simulink model "Aufgabe_13_simulink"  (Simulink 9.2)
settings: Solver=ode45  StartTime=0.0  StopTime=30  RelTol=1e-3  EnableMultiTasking=on
InitFcn:
  | Aufgabe_5_initFunction_Vorlage
StopFcn:
  | if Testen == 1
  | 
  | addpath('Check');
  | Aufgabe_5_Kontrolle;
  | 
  | end
undefined symbols (not defined in the file or in its folder): t_save
libraries: dspnetwork x4
settings Model: Creator=St  LastModifiedBy=danial
settings SolverCC: ZeroCrossAlgorithm=Adaptive
settings DataIOCC: SignalLoggingSaveFormat=Dataset
settings DebuggingCC: SolverPrmCheckMsg=warning  FcnCallInpInsideContextMsg=error
settings GRTTargetCC: CombineOutputUpdateFcns=on  GRTInterface=off
settings ConfigComp: CovSFcnEnable=off
settings CustomProperty: DataType=string  Value=0

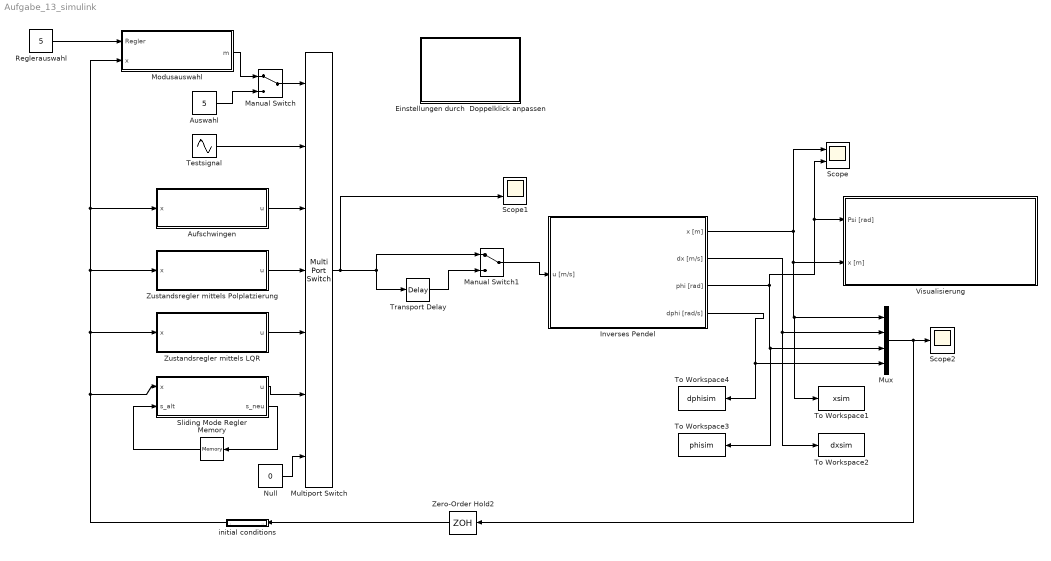
== system Aufgabe_13_simulink ==
  Aufschwingen : MATLAB Function  TreatAsAtomicUnit=on
  Auswahl : Constant  Value=5  SampleTime=-1
  Einstellungen durch  Doppelklick anpassen : MATLAB Function  InitFcn=tic  TreatAsAtomicUnit=on  mask{Auswahl=Bearbeiten}
      mask init:
      | maskStr = get_param(gcb,'Auswahl');
      | 
      | if strcmp(maskStr(1),'I')
      |      assignin('base','Testen',0)
      | else if strcmp(maskStr(1),'M')
      |         assignin('base','Testen',1)
      |     else
      |         assignin('base','Testen',2)
      |     end
      | end
  Inverses Pendel : Subsystem  TreatAsAtomicUnit=on  mask{x0=0, dx0=0.5, phi0=0, dphi0=0}
      mask prompts: x0 "Startposition Wagen [m]"; dx0 "Startgeschwindigkeit Wagen [m/s]"; phi0 "Startwinkel Pendel [rad]"; dphi0 "Startwinkelgeschwindigkeit Pendel [rad/s]"
  Manual Switch : ManualSwitch
  Manual Switch1 : ManualSwitch
  Memory : Memory  InitialCondition=-2
  Modusauswahl : MATLAB Function  TreatAsAtomicUnit=on
  Multiport Switch : MultiPortSwitch  Inputs=5  DataPortForDefault=Additional data port  DiagnosticForDefault=Warning
  Mux : Mux
  Null : Constant  Value=0  SampleTime=-1
  Reglerauswahl : Constant  Value=5  SampleTime=-1
  Scope : Scope  NumInputPorts=2
  Scope1 : Scope  NumInputPorts=2
  Scope2 : Scope
  Sliding Mode Regler : MATLAB Function  TreatAsAtomicUnit=on
  Testsignal : Sin  Amplitude=0.5  Frequency=6  SampleTime=0
  To Workspace1 : ToWorkspace  VariableName=xsim  SampleTime=t_save
  To Workspace2 : ToWorkspace  VariableName=dxsim  SampleTime=t_save
  To Workspace3 : ToWorkspace  VariableName=phisim  SampleTime=t_save
  To Workspace4 : ToWorkspace  VariableName=dphisim  SampleTime=t_save
  Transport Delay : TransportDelay  DelayTime=0.03
  Visualisierung : Subsystem
      mask init:
      | l_s = 0.5;              % Schienenlänge [m]
      settings: OpenFcn=|
      | !Pendel_Visualisierung_64bit\Pendel.blend.exe
      | !Pendel_Visualisierung_32bit\Pendel.blend.exe
  Zero-Order Hold2 : ZeroOrderHold  SampleTime=0.005
  Zustandsregler mittels LQR : MATLAB Function  TreatAsAtomicUnit=on
  Zustandsregler mittels Polplatzierung : MATLAB Function  TreatAsAtomicUnit=on
  initial conditions : Subsystem  mask{x0=0, dx0=0, phi0=pi, dphi0=0}
      mask prompts: x0 "Startposition Wagen [m]"; dx0 "Startgeschwindigkeit Wagen [m/s]"; phi0 "Startwinkel Pendel [rad]"; dphi0 "Startwinkelgeschwindigkeit Pendel [rad/s]"
  wires:
  Inverses Pendel/1(x [m]) -> Scope/1, To Workspace1/1, Mux/1, Visualisierung/2(x [m])
  Inverses Pendel/3(phi [rad]) -> Visualisierung/1(Psi [rad]), Scope/2, To Workspace3/1, Mux/3
  Null/1 -> Multiport Switch/7
  Testsignal/1 -> Multiport Switch/2
  Zustandsregler mittels Polplatzierung/1(u) -> Multiport Switch/4
  Inverses Pendel/2(dx [m/s]) -> To Workspace2/1, Mux/2
  Inverses Pendel/4(dphi [rad/s]) -> To Workspace4/1, Mux/4
  Zustandsregler mittels LQR/1(u) -> Multiport Switch/5
  Sliding Mode Regler/1(u) -> Multiport Switch/6
  Auswahl/1 -> Manual Switch/2
  Modusauswahl/1(m) -> Manual Switch/1
  Manual Switch/1 -> Multiport Switch/1
  Aufschwingen/1(u) -> Multiport Switch/3
  Reglerauswahl/1 -> Modusauswahl/1(Regler)
  initial conditions/1(.) -> Sliding Mode Regler/1(x), Zustandsregler mittels LQR/1(x), Aufschwingen/1(x), Modusauswahl/2(x), Zustandsregler mittels Polplatzierung/1(x)
  Mux/1 -> Zero-Order Hold2/1, Scope2/1
  Zero-Order Hold2/1 -> initial conditions/1(..)
  Sliding Mode Regler/2(s_neu) -> Memory/1
  Memory/1 -> Sliding Mode Regler/2(s_alt)
  Manual Switch1/1 -> Inverses Pendel/1(u [m/s])
  Transport Delay/1 -> Manual Switch1/2
  Multiport Switch/1 -> Transport Delay/1, Manual Switch1/1, Scope1/2

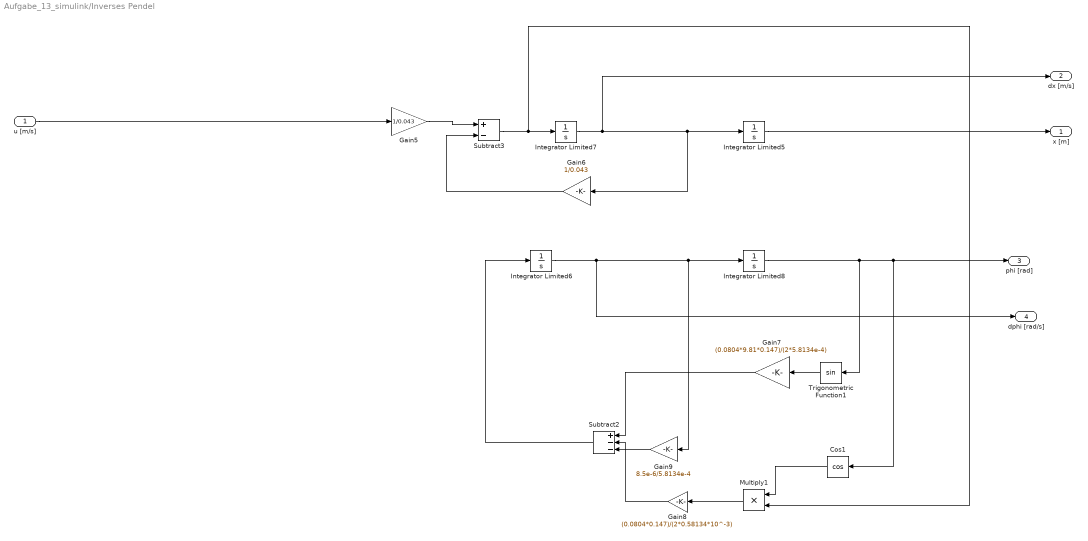
== system Aufgabe_13_simulink/Inverses Pendel ==
  u [m/s] : Inport
  Cos1 : Trigonometry  Operator=cos
  Gain5 : Gain  Gain=1/0.043
  Gain6 : Gain  Gain=1/0.043
  Gain7 : Gain  Gain=(0.0804*9.81*0.147)/(2*5.8134e-4)
  Gain8 : Gain  Gain=(0.0804*0.147)/(2*0.58134*10^-3)
  Gain9 : Gain  Gain=8.5e-6/5.8134e-4
  Integrator Limited5 : Integrator  InitialCondition=x0  LimitOutput=on  UpperSaturationLimit=0.25  LowerSaturationLimit=-0.25
  Integrator Limited6 : Integrator  InitialCondition=dphi0  UpperSaturationLimit=1  LowerSaturationLimit=0
  Integrator Limited7 : Integrator  InitialCondition=dx0  LimitOutput=on  UpperSaturationLimit=0.73  LowerSaturationLimit=-0.73
  Integrator Limited8 : Integrator  InitialCondition=phi0  UpperSaturationLimit=1  LowerSaturationLimit=0
  Multiply1 : Product
  Subtract2 : Sum  Inputs=+--
  Subtract3 : Sum  Inputs=+-
  Trigonometric Function1 : Trigonometry
  x [m] : Outport
  dx [m/s] : Outport  Port=2
  phi [rad] : Outport  Port=3
  dphi [rad/s] : Outport  Port=4
  wires:
  Integrator Limited8/1 -> Trigonometric Function1/1, phi [rad]/1, Cos1/1
  u [m/s]/1 -> Gain5/1
  Subtract3/1 -> Multiply1/2, Integrator Limited7/1
  Integrator Limited6/1 -> dphi [rad/s]/1, Integrator Limited8/1, Gain9/1
  Gain7/1 -> Subtract2/1
  Cos1/1 -> Multiply1/1
  Integrator Limited5/1 -> x [m]/1
  Subtract2/1 -> Integrator Limited6/1
  Gain8/1 -> Subtract2/2
  Trigonometric Function1/1 -> Gain7/1
  Gain5/1 -> Subtract3/1
  Gain6/1 -> Subtract3/2
  Multiply1/1 -> Gain8/1
  Gain9/1 -> Subtract2/3
  Integrator Limited7/1 -> dx [m/s]/1, Integrator Limited5/1, Gain6/1

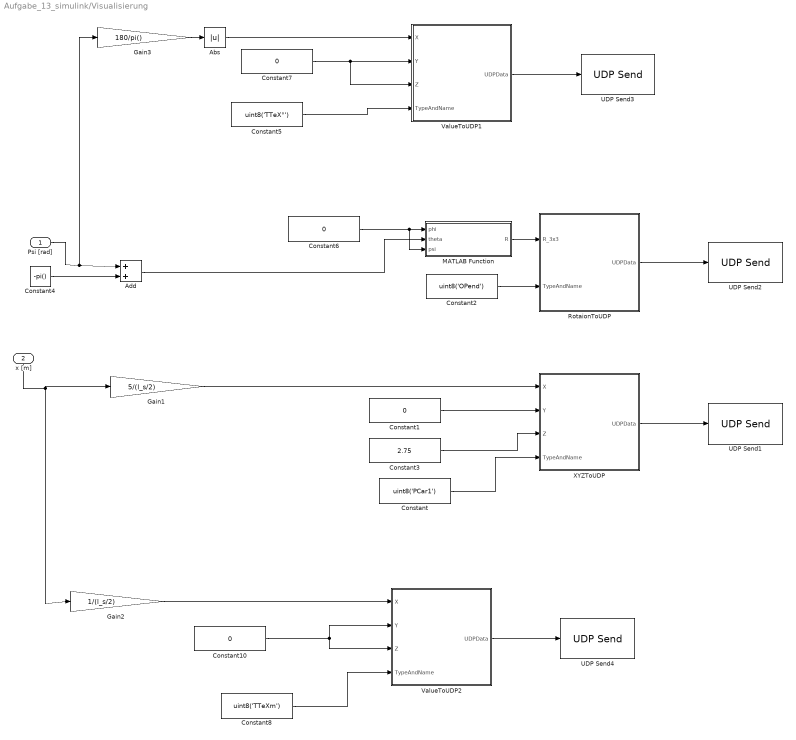
== system Aufgabe_13_simulink/Visualisierung ==
  Psi [rad] : Inport
  x [m] : Inport  Port=2
  Abs : Abs
  Add : Sum
  Constant : Constant  Value=uint8('PCar1')
  Constant{1,6..7,10} (4 alike) : Constant  Value=0
  Constant2 : Constant  Value=uint8('OPend')
  Constant3 : Constant  Value=2.75
  Constant4 : Constant  Value=-pi()
  Constant5 : Constant  Value=uint8('TTeX°')
  Constant8 : Constant  Value=uint8('TTeXm')
  Gain1 : Gain  Gain=5/(l_s/2)
  Gain2 : Gain  Gain=1/(l_s/2)
  Gain3 : Gain  Gain=180/pi()
  MATLAB Function : MATLAB Function  TreatAsAtomicUnit=on
  RotaionToUDP : Subsystem
  UDP Send{1..4} (4 alike) : dspnetwork/UDP Send  remoteURL='localhost'  remotePort=9999  localURL='0.0.0.0'  localPortSource=Automatically determine  localPort=-1  sampletime=-1  blockPlatform=WINDOWS  separateLengthPort=0
      settings: SourceProductName=DSP System Toolbox  SourceProductBaseCode=DS
  ValueToUDP1 : Subsystem
  ValueToUDP2 : Subsystem
  XYZToUDP : Subsystem
  wires:
  Constant2/1 -> RotaionToUDP/2(TypeAndName)
  XYZToUDP/1(UDPData) -> UDP Send1/1
  MATLAB Function/1(R) -> RotaionToUDP/1("R_3x3 ")
  Constant6/1 -> MATLAB Function/3(psi), MATLAB Function/1(phi)
  RotaionToUDP/1(UDPData) -> UDP Send2/1
  Constant/1 -> XYZToUDP/4(TypeAndName)
  Constant1/1 -> XYZToUDP/2(Y)
  Constant3/1 -> XYZToUDP/3(Z)
  Gain1/1 -> XYZToUDP/1(X)
  Add/1 -> MATLAB Function/2(theta)
  Constant4/1 -> Add/2
  ValueToUDP1/1(UDPData) -> UDP Send3/1
  Constant5/1 -> ValueToUDP1/4(TypeAndName)
  Constant7/1 -> ValueToUDP1/3(Z), ValueToUDP1/2(Y)
  Psi [rad]/1 -> Gain3/1, Add/1
  ValueToUDP2/1(UDPData) -> UDP Send4/1
  Constant8/1 -> ValueToUDP2/4(TypeAndName)
  x [m]/1 -> Gain2/1, Gain1/1
  Gain2/1 -> ValueToUDP2/1(X)
  Gain3/1 -> Abs/1
  Abs/1 -> ValueToUDP1/1(X)
  Constant10/1 -> ValueToUDP2/2(Y), ValueToUDP2/3(Z)

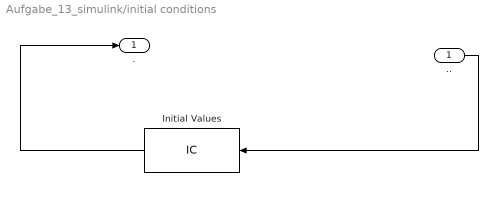
== system Aufgabe_13_simulink/initial conditions ==
  .. : Inport
  Initial Values : InitialCondition  Value=[x0 dx0 phi0 dphi0]
  . : Outport
  wires:
  ../1 -> Initial Values/1
  Initial Values/1 -> ./1

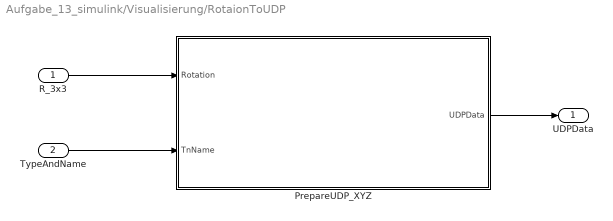
== system Aufgabe_13_simulink/Visualisierung/RotaionToUDP ==
  "R_3x3 " : Inport
  TypeAndName : Inport  Port=2
  PrepareUDP_XYZ : MATLAB Function  TreatAsAtomicUnit=on
  UDPData : Outport
  wires:
  TypeAndName/1 -> PrepareUDP_XYZ/2(TnName)
  "R_3x3 "/1 -> PrepareUDP_XYZ/1(Rotation)
  PrepareUDP_XYZ/1(UDPData) -> UDPData/1

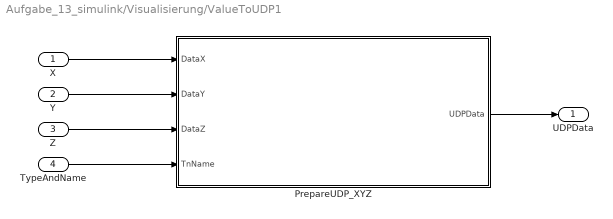
== system Aufgabe_13_simulink/Visualisierung/ValueToUDP1 ==
  X : Inport
  Y : Inport  Port=2
  Z : Inport  Port=3
  TypeAndName : Inport  Port=4
  PrepareUDP_XYZ : MATLAB Function  TreatAsAtomicUnit=on
  UDPData : Outport
  wires:
  Y/1 -> PrepareUDP_XYZ/2(DataY)
  Z/1 -> PrepareUDP_XYZ/3(DataZ)
  TypeAndName/1 -> PrepareUDP_XYZ/4(TnName)
  X/1 -> PrepareUDP_XYZ/1(DataX)
  PrepareUDP_XYZ/1(UDPData) -> UDPData/1

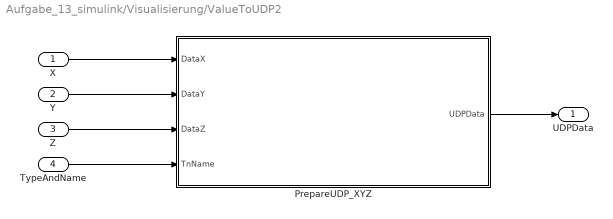
== system Aufgabe_13_simulink/Visualisierung/ValueToUDP2 ==
  X : Inport
  Y : Inport  Port=2
  Z : Inport  Port=3
  TypeAndName : Inport  Port=4
  PrepareUDP_XYZ : MATLAB Function  TreatAsAtomicUnit=on
  UDPData : Outport
  wires:
  Y/1 -> PrepareUDP_XYZ/2(DataY)
  Z/1 -> PrepareUDP_XYZ/3(DataZ)
  TypeAndName/1 -> PrepareUDP_XYZ/4(TnName)
  X/1 -> PrepareUDP_XYZ/1(DataX)
  PrepareUDP_XYZ/1(UDPData) -> UDPData/1

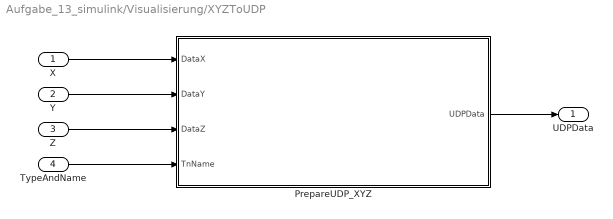
== system Aufgabe_13_simulink/Visualisierung/XYZToUDP ==
  X : Inport
  Y : Inport  Port=2
  Z : Inport  Port=3
  TypeAndName : Inport  Port=4
  PrepareUDP_XYZ : MATLAB Function  TreatAsAtomicUnit=on
  UDPData : Outport
  wires:
  Y/1 -> PrepareUDP_XYZ/2(DataY)
  Z/1 -> PrepareUDP_XYZ/3(DataZ)
  TypeAndName/1 -> PrepareUDP_XYZ/4(TnName)
  X/1 -> PrepareUDP_XYZ/1(DataX)
  PrepareUDP_XYZ/1(UDPData) -> UDPData/1

== matlab function Zustandsregler mittels Polplatzierung ==
  data: u output double; x input double
function u = Zustandsregler(x) %#codegen
%% Polvorgabe
K = [-0.3814,   -1.6067,   -2.8471,   -0.2415];
u = -K*x;

== matlab function Einstellungen durch Doppelklick anpassen ==
  settings: updateMethod=DISCRETE  sampleTime=0.1
function Auswahl


coder.extrinsic('tic');
coder.extrinsic('toc');
coder.extrinsic('drawnow');
coder.extrinsic('evalin');

Testen = 0;
Testen = evalin('base','Testen');

if Testen == 0

    t = 0;
    t = toc;
    while t < 0.1
    t = toc;
    drawnow;
    end
    tic;

end

== matlab function Zustandsregler mittels LQR ==
  data: u output double; x input double
function u = Zustandsregler_LQR(x) %#codegen

%% Implementierung des Zustandsreglers mit LQR
%K = [-0.0949,   -1.9733,   -2.7982,   -0.2800];
%K = [-0.9304,   -2.2265,   -3.3567,   -0.3359];
%K =[-0.8337,   -3.9484,   -6.6079,   -0.6612];
K =[-2.6537,   -3.0531,   -5.6334,   -0.5636];
%K = [-0.3489,   -4.6508,   -8.1286,   -0.8134];

u = -K*x;

== matlab function Sliding Mode Regler ==
  data: u output double; x input double; s_alt input double; s_neu output double
function [u,s_neu] = Sliding_Mode_Regler(x,s_alt) %#codegen

%% Auswahl des Schaltgesetzes für den Sliding-Mode-Regler

auswahl = 1;    % 1 ... mit sign-Funktion
                % 2 ... mit sat-Funktion

                
%% Definitionen und Initialisierung interner Variablen                 
% Speichert den Wert der Schaltfläche vom letzen Aufruf zur Behandlung des Falls s=0 der Signum-Funktion

if (s_alt == -2)   % Beim ersten Aufruf wird die Variable 0 initialisiert 
    s_alt = 0;
end

%% Regelungsnormalform Variabeln:
%Die letzte Zeile der Matriz A:

a_ll = [0,    2319,   99.38,  -23.27];

TR = [-0.0004,   -0.0000,   -0.0000,   -0.0000;
         0,   -0.0004,   -0.0000,   -0.0000;
         0,    0.0000,   -0.0042,   -0.0000;
         0,   -0.0000,   -0.0000,   -0.0042;
     ];
 %Zustände in Normalform
 x_n = TR*x;
 
 %% Slidingmode Regler
 
 %eta und lambda parameter
 eta = 0.02;
 lambda = 10;
 phi = 0.001;
 % berechnung von s und s_punkt
 s = x_n(4) + 3*lambda*x_n(3) + 3*lambda^2*x_n(2) + lambda^3*x_n(1);
 u_von_s_p = -3*lambda*x_n(4) - 3*lambda^2*x_n(3) - lambda^3*x_n(2) ...
     -a_ll(1)*x_n(1) - a_ll(2)*x_n(2) - a_ll(3)*x_n(3) - a_ll(4)*x_n(4);
 
 
 % sign funktion:
 if auswahl == 1
     if (s<0)
         sign_s = -1;       
     elseif( s>0)
         sign_s = 1;
     else % wenn s = 0 dann benutze s vom letzten zyklus um die vorzeichnen zu wechseln
         if(s_alt < 0)
             sign_s = 1;
         else
             sign_s = -1;
         end
     end
     u = u_von_s_p - eta*sign_s;
 else
     if (s < -phi)
        sat = -1;
    elseif (s > phi)
        sat = 1;
    else
        sat = s/phi;
     end
    u = u_von_s_p - eta*sat;
 end
 s_neu = s;

== matlab function Aufschwingen ==
  data: u output double; x input double
function u = Aufschwingen(x) %#codegen

%% Konstanten definieren

% Umrechnungsfaktor von deg in rad
DEG_ZU_RAD = pi/180;

% Wagengeschwindigkeit zum Aufschwingen [m/s]
AUFSCHWING_ACC = 0.2;


%% Umrechnung in reale Messgrößen: phi = (-180,180]
phi = x(3);
dphi = x(4);

phi = mod(phi,2*pi);

if (phi>pi) 
    phi = -2*pi+phi;
elseif(phi<-pi)
    phi = 2*pi+phi;
end


%% Implementierung des Aufschwingens

u = 0;

== matlab function Modusauswahl ==
  data: Regler input double; m output double; x input double
function m = Modusauswahl(Regler,x) %#codegen

%% Umrechnung in reale Messgrößen: phi = (-180,180]
phi = x(3);
dphi = x(4);

phi = mod(phi,2*pi);

if (phi>pi) 
    phi = -2*pi+phi;
elseif(phi<-pi)
    phi = 2*pi+phi;
end


%% Konstanten definieren

% Umrechnungsfaktor von deg in rad
DEG_ZU_RAD = pi/180;

% Winkelbereich, für den Regler aktiviert [rad]
PHI_REG_AKTIV = 20*DEG_ZU_RAD;

% Winkelgeschwindigkeitsbereich, für den Regler aktiv [rad/s]
DPHI_REG_AKTIV = 180*DEG_ZU_RAD;

% Winkelgeschwindigkeitsbereich, für den Aufschwingen aktiv [rad/s]
DPHI_AUF_AKTIV = 970*DEG_ZU_RAD;


%% Modusauswahl

if ((abs(phi) < PHI_REG_AKTIV) && (abs(dphi) < DPHI_REG_AKTIV))
    m = Regler; % Zustandsregler, LQR-Regler oder Sliding Mode Regler aktiv
elseif ((abs(phi) >= PHI_REG_AKTIV) && (abs(dphi) < DPHI_AUF_AKTIV))
    m = 2; % Aufschwingen aktiv
else
    m = 0; % Warten
end

== matlab function Visualisierung/MATLAB Function ==
  data: phi input double; R output double; theta input double; psi input double
function R = RotMatrix(phi, theta, psi)
cphi = cos(phi);
sphi = sin(phi);
ctheta  = cos(theta);
stheta  = sin(theta);
cpsi = cos(psi);
spsi = sin(psi);

R = [cpsi*ctheta -spsi*cphi+cpsi*stheta*sphi spsi*sphi+cpsi*cphi*stheta ; spsi*ctheta cpsi*cphi+sphi*stheta*spsi -cpsi*sphi+stheta*spsi*cphi ; -stheta ctheta*sphi ctheta*cphi ];

== matlab function Visualisierung/ValueToUDP1/PrepareUDP_XYZ ==
  data: DataX input double; DataY input double; DataZ input double; UDPData output uint8; TnName input double
function UDPData = XYZToBlenderUdpConversion(DataX,DataY,DataZ,TnName)
tx=typecast(single(DataX),'uint8')';
ty=typecast(single(DataY),'uint8')';
tz=typecast(single(DataZ),'uint8')';
UDPData=zeros(17,1,'uint8');
UDPData=[TnName;tx;ty;tz];

== matlab function Visualisierung/RotaionToUDP/PrepareUDP_XYZ ==
  data: Rotation input double; UDPData output uint8; TnName input double
function UDPData = RotationToBlenderUdpConversion(Rotation,TnName)
r1=typecast(single(Rotation(1,:)),'uint8')';
r2=typecast(single(Rotation(2,:)),'uint8')';
r3=typecast(single(Rotation(3,:)),'uint8')';
UDPData=zeros(41,1,'uint8');
UDPData=[TnName;r1;r2;r3];

== matlab function Visualisierung/XYZToUDP/PrepareUDP_XYZ ==
  data: DataX input double; DataY input double; DataZ input double; UDPData output uint8; TnName input double
function UDPData = XYZToBlenderUdpConversion(DataX,DataY,DataZ,TnName)
tx=typecast(single(DataX),'uint8')';
ty=typecast(single(DataY),'uint8')';
tz=typecast(single(DataZ),'uint8')';
UDPData=zeros(17,1,'uint8');
UDPData=[TnName;tx;ty;tz];

== matlab function Visualisierung/ValueToUDP2/PrepareUDP_XYZ ==
  data: DataX input double; DataY input double; DataZ input double; UDPData output uint8; TnName input double
function UDPData = XYZToBlenderUdpConversion(DataX,DataY,DataZ,TnName)
tx=typecast(single(DataX),'uint8')';
ty=typecast(single(DataY),'uint8')';
tz=typecast(single(DataZ),'uint8')';
UDPData=zeros(17,1,'uint8');
UDPData=[TnName;tx;ty;tz];
